simulink model "PegasusAutopilot"  (R2016a)
settings: Solver=ode4  StartTime=0.0  StopTime=inf  FixedStep=0.01  RelTol=1e-3
undefined symbols (not defined in the file): Ch, Cphi, Ctheta, CVt, degtorad, Kh, Kp, Kphi, Kpsi, Kq, Kr, Ktheta, KVt, tau, Ue
libraries: simulink x5
settings Model: PauseTimes=29  Creator=Marcelo Henrique  LastModifiedBy=Marcelo
settings SolverCC: AlgebraicLoopSolver=LineSearch
settings DataIOCC: LimitDataPoints=on  SaveFormat=Array
settings DebuggingCC: AlgebraicLoopMsg=none  UnderspecifiedInitializationDetection=Classic  MergeDetectMultiDrivingBlocksExec=none  StateNameClashWarn=warning
settings HardwareCC: ProdBitPerPointer=32  ProdLargestAtomicFloat=None  ProdIntDivRoundTo=Undefined  ProdEndianess=Unspecified  ProdWordSize=32  ProdHWDeviceType=32-bit Generic
settings ModelReferenceCC: PropagateSignalLabelsOutOfModel=off
settings ConfigComp: CovModelRefEnable=Off

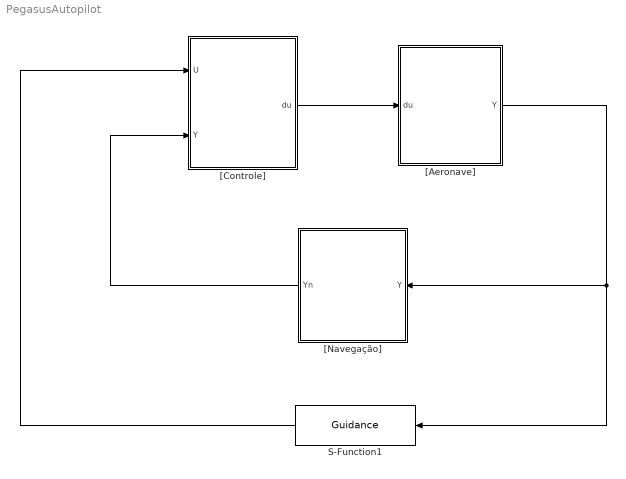
== system PegasusAutopilot ==
  S-Function1 : S-Function  FunctionName=Guidance  Parameters=WP, lambda  SFunctionDeploymentMode=off  EnableBusSupport=off
  "[Aeronave]" : Subsystem
  "[Controle]" : Subsystem
  "[Navegação]" : Subsystem
  wires:
  "[Navegação]"/1(Yn) -> "[Controle]"/2(Y)
  "[Controle]"/1(du) -> "[Aeronave]"/1(du)
  S-Function1/1 -> "[Controle]"/1(U)
  "[Aeronave]"/1(Y) -> "[Navegação]"/1(Y), S-Function1/1

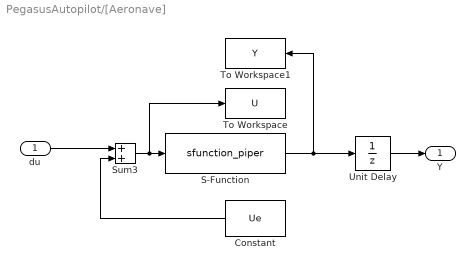
== system PegasusAutopilot/[Aeronave] ==
  du : Inport
  Constant : Constant  Value=Ue
  S-Function : S-Function  FunctionName=sfunction_piper  Parameters=par_gen,par_aero,par_prop, Xe  SFunctionDeploymentMode=off  EnableBusSupport=off
  Sum3 : Sum
  To Workspace : ToWorkspace  VariableName=U  SaveFormat=Timeseries  SampleTime=-1
  To Workspace1 : ToWorkspace  VariableName=Y  SaveFormat=Timeseries  SampleTime=-1
  Unit Delay : UnitDelay  SampleTime=-1
  Y : Outport
  wires:
  du/1 -> Sum3/1
  S-Function/1 -> To Workspace1/1, Unit Delay/1
  Constant/1 -> Sum3/2
  Sum3/1 -> To Workspace/1, S-Function/1
  Unit Delay/1 -> Y/1

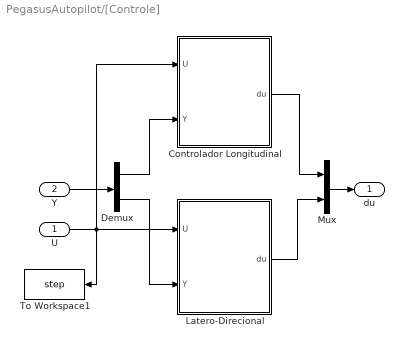
== system PegasusAutopilot/[Controle] ==
  U : Inport
  Y : Inport  Port=2
  Controlador Longitudinal : Subsystem
  Demux : Demux  Outputs=2
  Latero-Direcional : Subsystem
  Mux : Mux  Inputs=2
  To Workspace1 : ToWorkspace  VariableName=step  SaveFormat=Timeseries  SampleTime=-1
  du : Outport
  wires:
  Mux/1 -> du/1
  Controlador Longitudinal/1(du) -> Mux/1
  Latero-Direcional/1(du) -> Mux/2
  Y/1 -> Demux/1
  Demux/2 -> Latero-Direcional/2(Y)
  Demux/1 -> Controlador Longitudinal/2(Y)
  U/1 -> To Workspace1/1, Controlador Longitudinal/1(U), Latero-Direcional/1(U)

== system PegasusAutopilot/[Navegação] ==
  Y : Inport
  Latero-Direcional : Subsystem
  Longitudinal : Subsystem
  Mux : Mux  Inputs=2
  Yn : Outport
  wires:
  Y/1 -> Latero-Direcional/1(Y), Longitudinal/1(Y)
  Mux/1 -> Yn/1
  Longitudinal/1(Ylon) -> Mux/1
  Latero-Direcional/1(Ylat) -> Mux/2

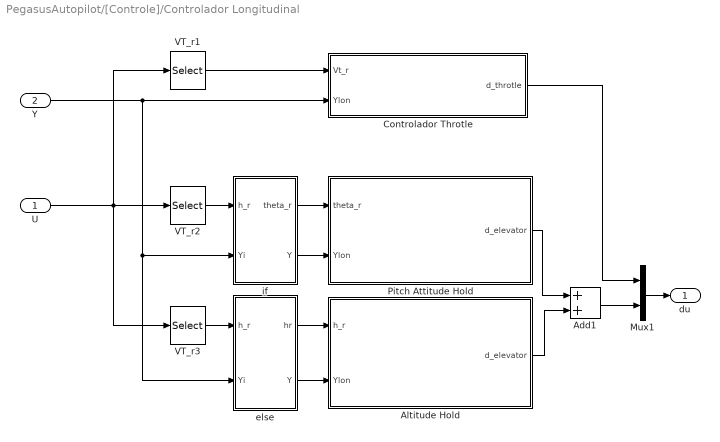
== system PegasusAutopilot/[Controle]/Controlador Longitudinal ==
  U : Inport
  Y : Inport  Port=2
  Add1 : Sum
  Altitude Hold : Subsystem
  Controlador Throtle : Subsystem
  Mux1 : Mux  Inputs=2
  Pitch Attitude Hold : Subsystem
  VT_r1 : Selector  InputPortWidth=3  IndexOptions=Index vector (dialog)  Indices=[1]  OutputSizes=1
  VT_r2 : Selector  InputPortWidth=3  IndexOptions=Index vector (dialog)  Indices=[2]  OutputSizes=1
  VT_r3 : Selector  InputPortWidth=3  IndexOptions=Index vector (dialog)  Indices=[2]  OutputSizes=1
  else : Subsystem
  if : Subsystem
  du : Outport
  wires:
  Pitch Attitude Hold/1(d_elevator) -> Add1/1
  Controlador Throtle/1(d_throtle) -> Mux1/1
  Altitude Hold/1(d_elevator) -> Add1/2
  Mux1/1 -> du/1
  if/2(Y) -> Pitch Attitude Hold/2(Ylon)
  Add1/1 -> Mux1/2
  if/1(theta_r) -> Pitch Attitude Hold/1(theta_r)
  else/2(Y) -> Altitude Hold/2(Ylon)
  else/1(hr) -> Altitude Hold/1(h_r)
  VT_r3/1 -> else/1(h_r)
  VT_r2/1 -> if/1(h_r)
  VT_r1/1 -> Controlador Throtle/1(Vt_r)
  Y/1 -> if/2(Yi), else/2(Yi), Controlador Throtle/2(Ylon)
  U/1 -> VT_r1/1, VT_r3/1, VT_r2/1

== system PegasusAutopilot/[Controle]/Latero-Direcional ==
  U : Inport
  Y : Inport  Port=2
  Controlador Ailerons : Subsystem
  Controlador Rudder : Subsystem
  Mux : Mux  Inputs=2
  VT_r1 : Selector  InputPortWidth=3  IndexOptions=Index vector (dialog)  Indices=[3]  OutputSizes=1
  du : Outport
  wires:
  Mux/1 -> du/1
  U/1 -> VT_r1/1
  Y/1 -> Controlador Ailerons/2(Yn), Controlador Rudder/1(Yn)
  Controlador Ailerons/1(d_aileron) -> Mux/1
  Controlador Rudder/1(d_rudder) -> Mux/2
  VT_r1/1 -> Controlador Ailerons/1(psi_r)

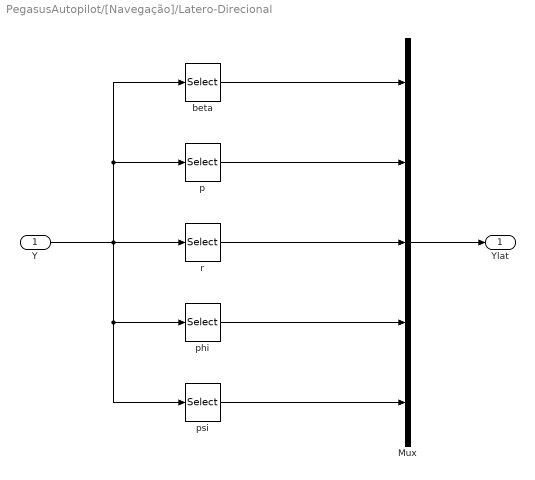
== system PegasusAutopilot/[Navegação]/Latero-Direcional ==
  Y : Inport
  Mux : Mux  Inputs=5
  beta : Selector  InputPortWidth=12  IndexOptions=Index vector (dialog)  Indices=[3]  OutputSizes=1
  p : Selector  InputPortWidth=12  IndexOptions=Index vector (dialog)  Indices=[4]  OutputSizes=1
  phi : Selector  InputPortWidth=12  IndexOptions=Index vector (dialog)  Indices=[7]  OutputSizes=1
  psi : Selector  InputPortWidth=12  IndexOptions=Index vector (dialog)  Indices=[9]  OutputSizes=1
  r : Selector  InputPortWidth=12  IndexOptions=Index vector (dialog)  Indices=[6]  OutputSizes=1
  Ylat : Outport
  wires:
  Y/1 -> psi/1, phi/1, beta/1, p/1, r/1
  beta/1 -> Mux/1
  phi/1 -> Mux/4
  psi/1 -> Mux/5
  p/1 -> Mux/2
  r/1 -> Mux/3
  Mux/1 -> Ylat/1

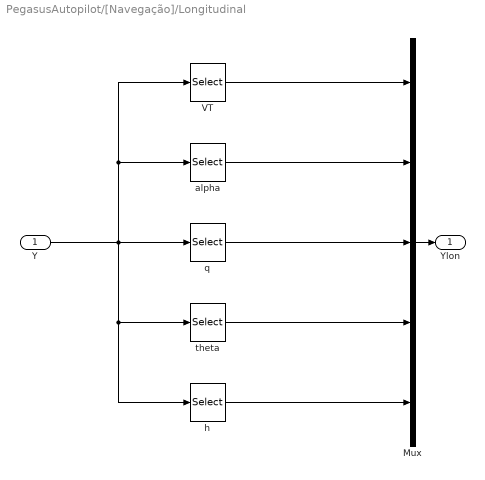
== system PegasusAutopilot/[Navegação]/Longitudinal ==
  Y : Inport
  Mux : Mux  Inputs=5
  VT : Selector  InputPortWidth=12  IndexOptions=Index vector (dialog)  Indices=[1]  OutputSizes=1
  alpha : Selector  InputPortWidth=12  IndexOptions=Index vector (dialog)  Indices=[2]  OutputSizes=1
  h : Selector  InputPortWidth=12  IndexOptions=Index vector (dialog)  Indices=[12]  OutputSizes=1
  q : Selector  InputPortWidth=12  IndexOptions=Index vector (dialog)  Indices=[5]  OutputSizes=1
  theta : Selector  InputPortWidth=12  IndexOptions=Index vector (dialog)  Indices=[8]  OutputSizes=1
  Ylon : Outport
  wires:
  VT/1 -> Mux/1
  q/1 -> Mux/3
  Y/1 -> h/1, theta/1, VT/1, alpha/1, q/1
  h/1 -> Mux/5
  alpha/1 -> Mux/2
  theta/1 -> Mux/4
  Mux/1 -> Ylon/1

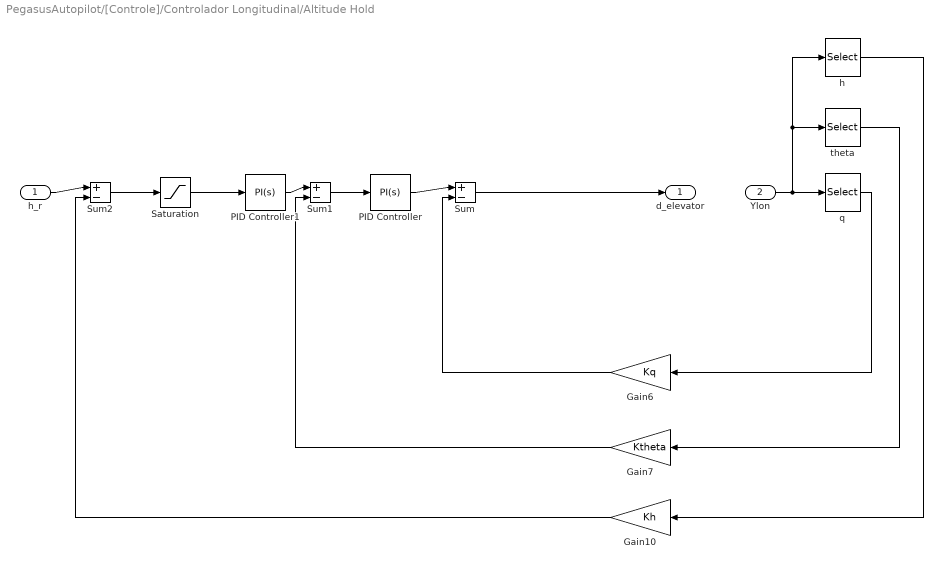
== system PegasusAutopilot/[Controle]/Controlador Longitudinal/Altitude Hold ==
  h_r : Inport
  Ylon : Inport  Port=2
  Gain10 : Gain  Gain=Kh
  Gain6 : Gain  Gain=Kq
  Gain7 : Gain  Gain=Ktheta
  PID Controller : simulink/Continuous/PID Controller  Controller=PI  TimeDomain=Continuous-time  SampleTime=-1  IntegratorMethod=Forward Euler  FilterMethod=Forward Euler  Form=Parallel  UseFilter=on  ControllerParametersSource=internal  P=Ctheta.Kp  I=Ctheta.Ki  D=0  N=100  InitialConditionSource=internal  InitialConditionForIntegrator=0  InitialConditionForFilter=0  ExternalReset=none  LimitOutput=off  UpperSaturationLimit=inf  LowerSaturationLimit=-inf  LinearizeAsGain=on  AntiWindupMode=none  Kb=1  TrackingMode=off  Kt=1  PParamMin=[]  PParamMax=[]  IParamMin=[]  IParamMax=[]  DParamMin=[]  DParamMax=[]  NParamMin=[]  NParamMax=[]  KbParamMin=[]  KbParamMax=[]  KtParamMin=[]  KtParamMax=[]  POutMin=[]  POutMax=[]  IOutMin=[]  IOutMax=[]  DOutMin=[]  DOutMax=[]  NOutMin=[]  NOutMax=[]  KbOutMin=[]  KbOutMax=[]  KtOutMin=[]  KtOutMax=[]  IntegratorOutMin=[]  IntegratorOutMax=[]  FilterOutMin=[]  FilterOutMax=[]  SumOutMin=[]  SumOutMax=[]  SumI1OutMin=[]  SumI1OutMax=[]  SumI2OutMin=[]  SumI2OutMax=[]  SumI3OutMin=[]  SumI3OutMax=[]  SumDOutMin=[]  SumDOutMax=[]  SaturationOutMin=[]  SaturationOutMax=[]  IntegratorContinuousStateAttributes=''  IntegratorStateMustResolveToSignalObject=off  IntegratorRTWStateStorageClass=Auto  FilterContinuousStateAttributes=''  FilterStateMustResolveToSignalObject=off  FilterRTWStateStorageClass=Auto  DifferentiatorICPrevScaledInput=0  DifferentiatorOutMin=[]  DifferentiatorOutMax=[]
  PID Controller1 : simulink/Continuous/PID Controller  Controller=PI  TimeDomain=Continuous-time  SampleTime=-1  IntegratorMethod=Forward Euler  FilterMethod=Forward Euler  Form=Parallel  UseFilter=on  ControllerParametersSource=internal  P=Ch.Kp  I=Ch.Ki  D=0  N=100  InitialConditionSource=internal  InitialConditionForIntegrator=0  InitialConditionForFilter=0  ExternalReset=none  LimitOutput=off  UpperSaturationLimit=inf  LowerSaturationLimit=-inf  LinearizeAsGain=on  AntiWindupMode=none  Kb=1  TrackingMode=off  Kt=1  PParamMin=[]  PParamMax=[]  IParamMin=[]  IParamMax=[]  DParamMin=[]  DParamMax=[]  NParamMin=[]  NParamMax=[]  KbParamMin=[]  KbParamMax=[]  KtParamMin=[]  KtParamMax=[]  POutMin=[]  POutMax=[]  IOutMin=[]  IOutMax=[]  DOutMin=[]  DOutMax=[]  NOutMin=[]  NOutMax=[]  KbOutMin=[]  KbOutMax=[]  KtOutMin=[]  KtOutMax=[]  IntegratorOutMin=[]  IntegratorOutMax=[]  FilterOutMin=[]  FilterOutMax=[]  SumOutMin=[]  SumOutMax=[]  SumI1OutMin=[]  SumI1OutMax=[]  SumI2OutMin=[]  SumI2OutMax=[]  SumI3OutMin=[]  SumI3OutMax=[]  SumDOutMin=[]  SumDOutMax=[]  SaturationOutMin=[]  SaturationOutMax=[]  IntegratorContinuousStateAttributes=''  IntegratorStateMustResolveToSignalObject=off  IntegratorRTWStateStorageClass=Auto  FilterContinuousStateAttributes=''  FilterStateMustResolveToSignalObject=off  FilterRTWStateStorageClass=Auto  DifferentiatorICPrevScaledInput=0  DifferentiatorOutMin=[]  DifferentiatorOutMax=[]
  Saturation : Saturate  UpperLimit=+5.0  LowerLimit=-5.0
  Sum : Sum  Inputs=|+-
  Sum1 : Sum  Inputs=|+-
  Sum2 : Sum  Inputs=|+-
  h : Selector  InputPortWidth=5  IndexOptions=Index vector (dialog)  Indices=[5]  OutputSizes=1
  q : Selector  InputPortWidth=5  IndexOptions=Index vector (dialog)  Indices=[3]  OutputSizes=1
  theta : Selector  InputPortWidth=5  IndexOptions=Index vector (dialog)  Indices=[4]  OutputSizes=1
  d_elevator : Outport
  wires:
  Gain6/1 -> Sum/2
  Gain7/1 -> Sum1/2
  PID Controller/1 -> Sum/1
  Sum1/1 -> PID Controller/1
  PID Controller1/1 -> Sum1/1
  Gain10/1 -> Sum2/2
  Sum2/1 -> Saturation/1
  theta/1 -> Gain7/1
  q/1 -> Gain6/1
  Ylon/1 -> theta/1, h/1, q/1
  h/1 -> Gain10/1
  Sum/1 -> d_elevator/1
  h_r/1 -> Sum2/1
  Saturation/1 -> PID Controller1/1

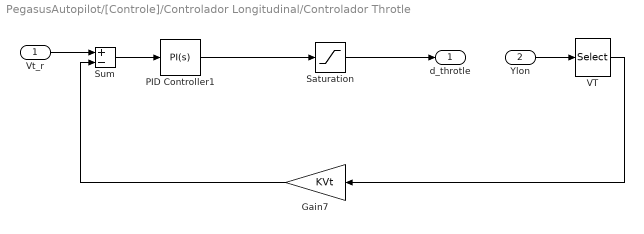
== system PegasusAutopilot/[Controle]/Controlador Longitudinal/Controlador Throtle ==
  Vt_r : Inport
  Ylon : Inport  Port=2
  Gain7 : Gain  Gain=KVt
  PID Controller1 : simulink/Continuous/PID Controller  Controller=PI  TimeDomain=Continuous-time  SampleTime=-1  IntegratorMethod=Forward Euler  FilterMethod=Forward Euler  Form=Parallel  UseFilter=on  ControllerParametersSource=internal  P=CVt.Kp  I=CVt.Ki  D=0  N=100  InitialConditionSource=internal  InitialConditionForIntegrator=0  InitialConditionForFilter=0  ExternalReset=none  LimitOutput=off  UpperSaturationLimit=inf  LowerSaturationLimit=-inf  LinearizeAsGain=on  AntiWindupMode=none  Kb=1  TrackingMode=off  Kt=1  PParamMin=[]  PParamMax=[]  IParamMin=[]  IParamMax=[]  DParamMin=[]  DParamMax=[]  NParamMin=[]  NParamMax=[]  KbParamMin=[]  KbParamMax=[]  KtParamMin=[]  KtParamMax=[]  POutMin=[]  POutMax=[]  IOutMin=[]  IOutMax=[]  DOutMin=[]  DOutMax=[]  NOutMin=[]  NOutMax=[]  KbOutMin=[]  KbOutMax=[]  KtOutMin=[]  KtOutMax=[]  IntegratorOutMin=[]  IntegratorOutMax=[]  FilterOutMin=[]  FilterOutMax=[]  SumOutMin=[]  SumOutMax=[]  SumI1OutMin=[]  SumI1OutMax=[]  SumI2OutMin=[]  SumI2OutMax=[]  SumI3OutMin=[]  SumI3OutMax=[]  SumDOutMin=[]  SumDOutMax=[]  SaturationOutMin=[]  SaturationOutMax=[]  IntegratorContinuousStateAttributes=''  IntegratorStateMustResolveToSignalObject=off  IntegratorRTWStateStorageClass=Auto  FilterContinuousStateAttributes=''  FilterStateMustResolveToSignalObject=off  FilterRTWStateStorageClass=Auto  DifferentiatorICPrevScaledInput=0  DifferentiatorOutMin=[]  DifferentiatorOutMax=[]
  Saturation : Saturate  UpperLimit=1  LowerLimit=-Ue(1)
  Sum : Sum  Inputs=+-
  VT : Selector  InputPortWidth=5  IndexOptions=Index vector (dialog)  Indices=1  OutputSizes=1
  d_throtle : Outport
  wires:
  Sum/1 -> PID Controller1/1
  Vt_r/1 -> Sum/1
  Ylon/1 -> VT/1
  VT/1 -> Gain7/1
  Gain7/1 -> Sum/2
  PID Controller1/1 -> Saturation/1
  Saturation/1 -> d_throtle/1

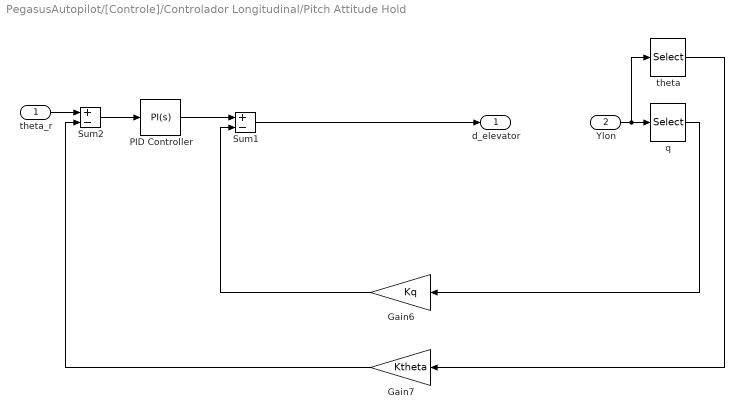
== system PegasusAutopilot/[Controle]/Controlador Longitudinal/Pitch Attitude Hold ==
  theta_r : Inport
  Ylon : Inport  Port=2
  Gain6 : Gain  Gain=Kq
  Gain7 : Gain  Gain=Ktheta
  PID Controller : simulink/Continuous/PID Controller  Controller=PI  TimeDomain=Continuous-time  SampleTime=-1  IntegratorMethod=Forward Euler  FilterMethod=Forward Euler  Form=Parallel  UseFilter=on  ControllerParametersSource=internal  P=Ctheta.Kp  I=Ctheta.Ki  D=0  N=100  InitialConditionSource=internal  InitialConditionForIntegrator=0  InitialConditionForFilter=0  ExternalReset=none  LimitOutput=off  UpperSaturationLimit=inf  LowerSaturationLimit=-inf  LinearizeAsGain=on  AntiWindupMode=none  Kb=1  TrackingMode=off  Kt=1  PParamMin=[]  PParamMax=[]  IParamMin=[]  IParamMax=[]  DParamMin=[]  DParamMax=[]  NParamMin=[]  NParamMax=[]  KbParamMin=[]  KbParamMax=[]  KtParamMin=[]  KtParamMax=[]  POutMin=[]  POutMax=[]  IOutMin=[]  IOutMax=[]  DOutMin=[]  DOutMax=[]  NOutMin=[]  NOutMax=[]  KbOutMin=[]  KbOutMax=[]  KtOutMin=[]  KtOutMax=[]  IntegratorOutMin=[]  IntegratorOutMax=[]  FilterOutMin=[]  FilterOutMax=[]  SumOutMin=[]  SumOutMax=[]  SumI1OutMin=[]  SumI1OutMax=[]  SumI2OutMin=[]  SumI2OutMax=[]  SumI3OutMin=[]  SumI3OutMax=[]  SumDOutMin=[]  SumDOutMax=[]  SaturationOutMin=[]  SaturationOutMax=[]  IntegratorContinuousStateAttributes=''  IntegratorStateMustResolveToSignalObject=off  IntegratorRTWStateStorageClass=Auto  FilterContinuousStateAttributes=''  FilterStateMustResolveToSignalObject=off  FilterRTWStateStorageClass=Auto  DifferentiatorICPrevScaledInput=0  DifferentiatorOutMin=[]  DifferentiatorOutMax=[]
  Sum1 : Sum  Inputs=+-
  Sum2 : Sum  Inputs=+-
  q : Selector  InputPortWidth=5  IndexOptions=Index vector (dialog)  Indices=[3]  OutputSizes=1
  theta : Selector  InputPortWidth=5  IndexOptions=Index vector (dialog)  Indices=[4]  OutputSizes=1
  d_elevator : Outport
  wires:
  theta/1 -> Gain7/1
  q/1 -> Gain6/1
  Gain6/1 -> Sum1/2
  Gain7/1 -> Sum2/2
  PID Controller/1 -> Sum1/1
  Sum2/1 -> PID Controller/1
  Ylon/1 -> theta/1, q/1
  Sum1/1 -> d_elevator/1
  theta_r/1 -> Sum2/1

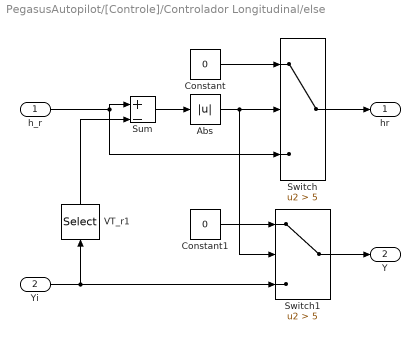
== system PegasusAutopilot/[Controle]/Controlador Longitudinal/else ==
  h_r : Inport
  Yi : Inport  Port=2
  Abs : Abs  ZeroCross=off
  Constant : Constant  Value=0
  Constant1 : Constant  Value=0
  Sum : Sum  Inputs=|+-
  Switch : Switch  Criteria=u2 > Threshold  Threshold=5  ZeroCross=off
  Switch1 : Switch  Criteria=u2 > Threshold  Threshold=5  ZeroCross=off
  VT_r1 : Selector  InputPortWidth=5  IndexOptions=Index vector (dialog)  Indices=[5]  OutputSizes=1
  hr : Outport
  Y : Outport  Port=2
  wires:
  Abs/1 -> Switch1/2, Switch/2
  Yi/1 -> Switch1/3, VT_r1/1
  Switch/1 -> hr/1
  Sum/1 -> Abs/1
  Switch1/1 -> Y/1
  Constant/1 -> Switch/1
  Constant1/1 -> Switch1/1
  h_r/1 -> Sum/1, Switch/3
  VT_r1/1 -> Sum/2

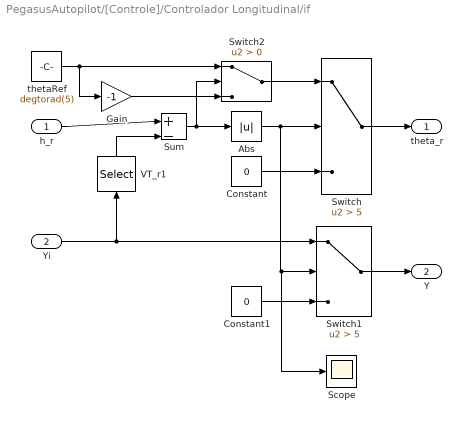
== system PegasusAutopilot/[Controle]/Controlador Longitudinal/if ==
  h_r : Inport
  Yi : Inport  Port=2
  Abs : Abs  ZeroCross=off
  Constant : Constant  Value=0
  Constant1 : Constant  Value=0
  Gain : Gain  Gain=-1
  Scope : Scope
  Sum : Sum  Inputs=|+-
  Switch : Switch  Criteria=u2 > Threshold  Threshold=5  ZeroCross=off
  Switch1 : Switch  Criteria=u2 > Threshold  Threshold=5  ZeroCross=off
  Switch2 : Switch  Criteria=u2 > Threshold  ZeroCross=off
  VT_r1 : Selector  InputPortWidth=5  IndexOptions=Index vector (dialog)  Indices=[5]  OutputSizes=1
  thetaRef : Constant  Value=degtorad(5)
  theta_r : Outport
  Y : Outport  Port=2
  wires:
  Abs/1 -> Scope/1, Switch1/2, Switch/2
  Switch/1 -> theta_r/1
  h_r/1 -> Sum/1
  Switch1/1 -> Y/1
  Constant/1 -> Switch/3
  Yi/1 -> VT_r1/1, Switch1/1
  Constant1/1 -> Switch1/3
  Gain/1 -> Switch2/3
  thetaRef/1 -> Gain/1, Switch2/1
  Switch2/1 -> Switch/1
  VT_r1/1 -> Sum/2
  Sum/1 -> Switch2/2, Abs/1

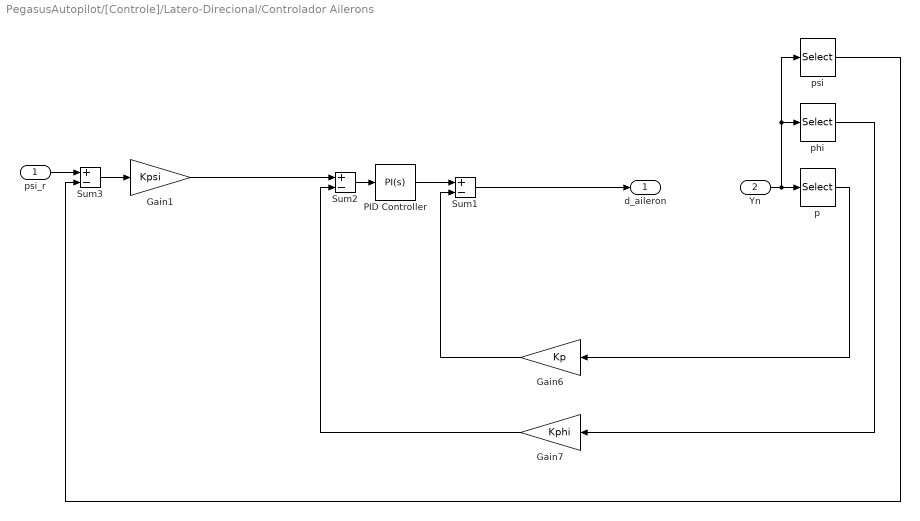
== system PegasusAutopilot/[Controle]/Latero-Direcional/Controlador Ailerons ==
  psi_r : Inport
  Yn : Inport  Port=2
  Gain1 : Gain  Gain=Kpsi
  Gain6 : Gain  Gain=Kp
  Gain7 : Gain  Gain=Kphi
  PID Controller : simulink/Continuous/PID Controller  Controller=PI  TimeDomain=Continuous-time  SampleTime=-1  IntegratorMethod=Forward Euler  FilterMethod=Forward Euler  Form=Parallel  UseFilter=on  ControllerParametersSource=internal  P=Cphi.Kp  I=Cphi.Ki  D=0  N=100  InitialConditionSource=internal  InitialConditionForIntegrator=0  InitialConditionForFilter=0  ExternalReset=none  LimitOutput=off  UpperSaturationLimit=inf  LowerSaturationLimit=-inf  LinearizeAsGain=on  AntiWindupMode=none  Kb=1  TrackingMode=off  Kt=1  PParamMin=[]  PParamMax=[]  IParamMin=[]  IParamMax=[]  DParamMin=[]  DParamMax=[]  NParamMin=[]  NParamMax=[]  KbParamMin=[]  KbParamMax=[]  KtParamMin=[]  KtParamMax=[]  POutMin=[]  POutMax=[]  IOutMin=[]  IOutMax=[]  DOutMin=[]  DOutMax=[]  NOutMin=[]  NOutMax=[]  KbOutMin=[]  KbOutMax=[]  KtOutMin=[]  KtOutMax=[]  IntegratorOutMin=[]  IntegratorOutMax=[]  FilterOutMin=[]  FilterOutMax=[]  SumOutMin=[]  SumOutMax=[]  SumI1OutMin=[]  SumI1OutMax=[]  SumI2OutMin=[]  SumI2OutMax=[]  SumI3OutMin=[]  SumI3OutMax=[]  SumDOutMin=[]  SumDOutMax=[]  SaturationOutMin=[]  SaturationOutMax=[]  IntegratorContinuousStateAttributes=''  IntegratorStateMustResolveToSignalObject=off  IntegratorRTWStateStorageClass=Auto  FilterContinuousStateAttributes=''  FilterStateMustResolveToSignalObject=off  FilterRTWStateStorageClass=Auto  DifferentiatorICPrevScaledInput=0  DifferentiatorOutMin=[]  DifferentiatorOutMax=[]
  Sum1 : Sum  Inputs=+-
  Sum2 : Sum  Inputs=+-
  Sum3 : Sum  Inputs=+-
  p : Selector  InputPortWidth=5  IndexOptions=Index vector (dialog)  Indices=[2]  OutputSizes=1
  phi : Selector  InputPortWidth=5  IndexOptions=Index vector (dialog)  Indices=[4]  OutputSizes=1
  psi : Selector  InputPortWidth=5  IndexOptions=Index vector (dialog)  Indices=[5]  OutputSizes=1
  d_aileron : Outport
  wires:
  phi/1 -> Gain7/1
  p/1 -> Gain6/1
  Gain6/1 -> Sum1/2
  Gain7/1 -> Sum2/2
  PID Controller/1 -> Sum1/1
  Sum2/1 -> PID Controller/1
  Yn/1 -> psi/1, phi/1, p/1
  Sum1/1 -> d_aileron/1
  psi/1 -> Sum3/2
  psi_r/1 -> Sum3/1
  Sum3/1 -> Gain1/1
  Gain1/1 -> Sum2/1

== system PegasusAutopilot/[Controle]/Latero-Direcional/Controlador Rudder ==
  Yn : Inport
  Gain6 : Gain  Gain=Kr
  Sum1 : Sum  Inputs=+-
  Washout Filter : TransferFcn  Numerator=[tau 0]  Denominator=[tau 1]
  r : Selector  InputPortWidth=5  IndexOptions=Index vector (dialog)  Indices=[3]  OutputSizes=1
  r_r : Constant  Value=0
  d_rudder : Outport
  wires:
  r/1 -> Washout Filter/1
  Gain6/1 -> Sum1/2
  r_r/1 -> Sum1/1
  Yn/1 -> r/1
  Sum1/1 -> d_rudder/1
  Washout Filter/1 -> Gain6/1
